simulink model "LPVattitudeLQRTracking"  (R2024b)
settings: Solver=ode45  StartTime=0.0  StopTime=tf  RelTol=1e-3
values from neighbouring files (symbols this model uses):
  gamma1_initial = deg2rad(0)    [CMG_Spacecraft_Attitude_Control.m]
  gamma2_initial = deg2rad(90)    [CMG_Spacecraft_Attitude_Control.m]
  p1 = linspace(gamma1_min,gamma1_max,gamma1_points)    [CMG_Spacecraft_Attitude_Control.m]
  p2 = linspace(gamma2_min,gamma2_max,gamma2_points)    [CMG_Spacecraft_Attitude_Control.m]
undefined symbols (not defined in the file or in its folder): K11, K12, K13, K14, K15, K16, K21, K22, K23, K24, K25, K26
libraries: simulink_extras x4, cstblocks x1
settings Model: PacingRate=1000  Creator=lanhi  LastModifiedBy=lanhi

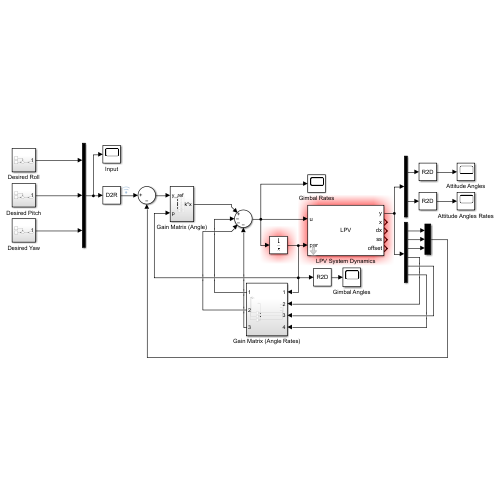
[thumbnail: Simulink's stored preview of the top-level diagram]
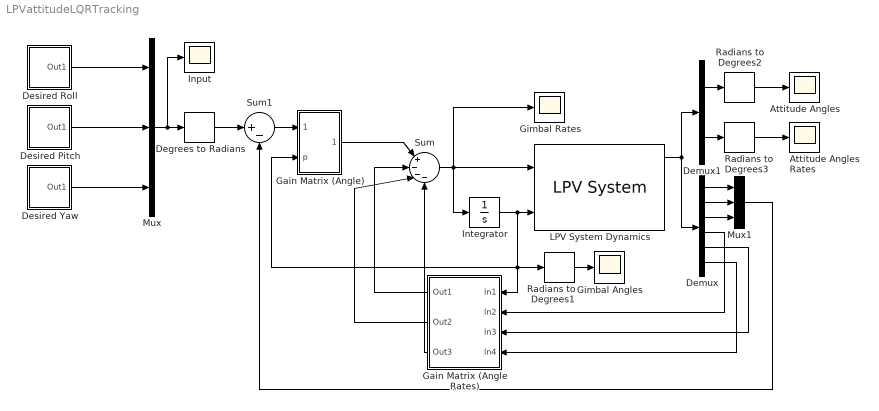
== system LPVattitudeLQRTracking ==
  Attitude Angles : Scope
  Attitude Angles Rates : Scope
  Degrees to Radians : simulink_extras/Transformations/Degrees to Radians
  Demux : Demux  Outputs=6
  Demux1 : Demux  Outputs=2
  Desired Pitch : Subsystem
  Desired Roll : Subsystem
  Desired Yaw : Subsystem
  Gain Matrix (Angle Rates) : Subsystem
  Gain Matrix (Angle) : Subsystem
  Gimbal Angles : Scope
  Gimbal Rates : Scope
  Input : Scope
  Integrator : Integrator  InitialCondition=[gamma1_initial,gamma2_initial]
  LPV System Dynamics : cstblocks/Linear Parameter Varying/LPV System  sys=ICs  InitialConditionSource=internal  InitialCondition=[deg2rad(0) deg2rad(0) deg2rad(0) deg2rad(0) deg2rad(0) deg2rad(0)]  opSpecOption=Specify offsets as double arrays  uOffset=0  yOffset=0  xOffset=0  opEquilOption=on  dxOffset=4  AFixed=false  BFixed=false  CFixed=false  DFixed=false  uDelayFixed=false  yDelayFixed=false  iDelayFixed=false  sysFixedOption=First model in state-space array  sysFixed=[]  IMethod=Linear  EMethod=Clip  IndexSearch=Binary search  IndexBegin=on  OutputX=on  OutputXdot=on  OutputLTI=on  OutputOP=on  DataType=double  InitBufferSize=1024  FixedBuffer=off  SimMode=Interpreted execution  Offset=struct
  Mux : Mux  Inputs=3
  Mux1 : Mux  Inputs=3
  Radians to Degrees1 : simulink_extras/Transformations/Radians to Degrees
  Radians to Degrees2 : simulink_extras/Transformations/Radians to Degrees
  Radians to Degrees3 : simulink_extras/Transformations/Radians to Degrees
  Sum : Sum  Inputs=|+---
  Sum1 : Sum  Inputs=|+-
  wires:
  Radians to Degrees1/1 -> Gimbal Angles/1
  LPV System Dynamics/1 -> Demux1/1, Demux/1
  Demux/1 -> Mux1/1
  Demux/2 -> Mux1/2
  Integrator/1 -> Gain Matrix (Angle Rates)/1(In1), Gain Matrix (Angle)/2(p), Radians to Degrees1/1, LPV System Dynamics/2
  Sum/1 -> Integrator/1, Gimbal Rates/1, LPV System Dynamics/1
  Gain Matrix (Angle)/1(k*x) -> Sum/1
  Mux/1 -> Degrees to Radians/1, Input/1
  Demux/3 -> Mux1/3
  Demux1/2 -> Radians to Degrees3/1
  Degrees to Radians/1 -> Sum1/1
  Sum1/1 -> Gain Matrix (Angle)/1(y_ref)
  Demux1/1 -> Radians to Degrees2/1
  Radians to Degrees2/1 -> Attitude Angles/1
  Radians to Degrees3/1 -> Attitude Angles Rates/1
  Mux1/1 -> Sum1/2
  Demux/4 -> Gain Matrix (Angle Rates)/2(In2)
  Demux/5 -> Gain Matrix (Angle Rates)/3(In3)
  Demux/6 -> Gain Matrix (Angle Rates)/4(In4)
  Gain Matrix (Angle Rates)/1(Out1) -> Sum/2
  Gain Matrix (Angle Rates)/2(Out2) -> Sum/3
  Gain Matrix (Angle Rates)/3(Out3) -> Sum/4
  Desired Roll/1(Out1) -> Mux/1
  Desired Pitch/1(Out1) -> Mux/2
  Desired Yaw/1(Out1) -> Mux/3

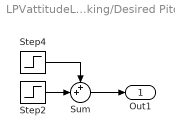
== system LPVattitudeLQRTracking/Desired Pitch ==
  Step2 : Step  Time=5  After=0  SampleTime=0
  Step4 : Step  After=0  SampleTime=0
  Sum : Sum  Inputs=++|
  Out1 : Outport
  wires:
  Step2/1 -> Sum/2
  Step4/1 -> Sum/1
  Sum/1 -> Out1/1

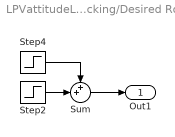
== system LPVattitudeLQRTracking/Desired Roll ==
  Step2 : Step  Time=5000  After=-15  SampleTime=0
  Step4 : Step  Time=1000  After=15  SampleTime=0
  Sum : Sum  Inputs=++|
  Out1 : Outport
  wires:
  Step2/1 -> Sum/2
  Step4/1 -> Sum/1
  Sum/1 -> Out1/1

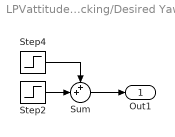
== system LPVattitudeLQRTracking/Desired Yaw ==
  Step2 : Step  Time=5  After=0  SampleTime=0
  Step4 : Step  After=0  SampleTime=0
  Sum : Sum  Inputs=++|
  Out1 : Outport
  wires:
  Step2/1 -> Sum/2
  Step4/1 -> Sum/1
  Sum/1 -> Out1/1

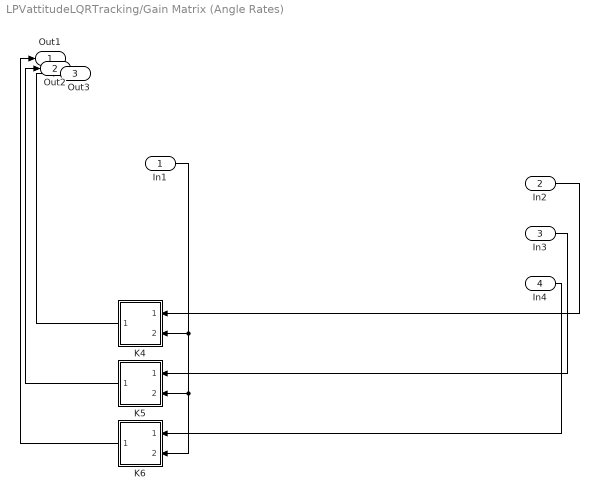
== system LPVattitudeLQRTracking/Gain Matrix (Angle Rates) ==
  In1 : Inport
  In2 : Inport  Port=2
  In3 : Inport  Port=3
  In4 : Inport  Port=4
  K4 : Subsystem
  K5 : Subsystem
  K6 : Subsystem
  Out1 : Outport
  Out2 : Outport  Port=2
  Out3 : Outport  Port=3
  wires:
  In2/1 -> K4/1(In1)
  K5/1(Out1) -> Out2/1
  In1/1 -> K6/2(In2), K5/2(In2), K4/2(In2)
  K6/1(Out1) -> Out1/1
  In4/1 -> K6/1(In1)
  K4/1(Out1) -> Out3/1
  In3/1 -> K5/1(In1)

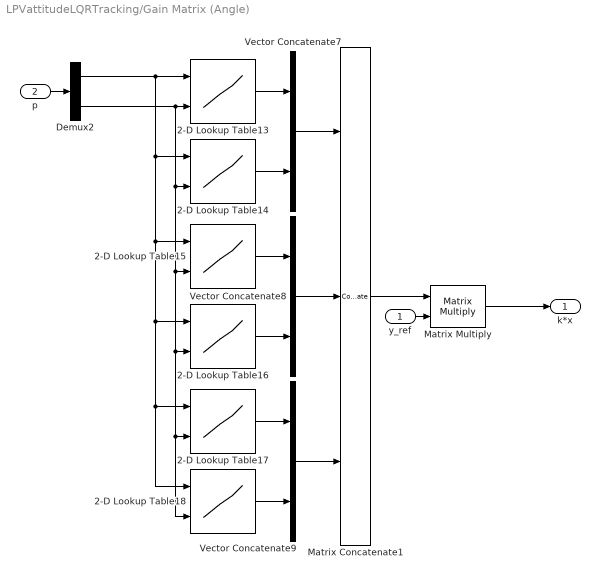
== system LPVattitudeLQRTracking/Gain Matrix (Angle) ==
  y_ref : Inport
  p : Inport  Port=2
  2-D Lookup Table13 : Lookup_n-D  BreakpointsForDimension1=p1  BreakpointsForDimension2=p2  Table=K11  InternalRulePriority=Speed  RndMeth=Simplest
      settings: InputPortMap=u0,u1
  2-D Lookup Table14 : Lookup_n-D  BreakpointsForDimension1=p1  BreakpointsForDimension2=p2  Table=K21  InternalRulePriority=Speed  RndMeth=Simplest
      settings: InputPortMap=u0,u1
  2-D Lookup Table15 : Lookup_n-D  BreakpointsForDimension1=p1  BreakpointsForDimension2=p2  Table=K12  InternalRulePriority=Speed  RndMeth=Simplest
      settings: InputPortMap=u0,u1
  2-D Lookup Table16 : Lookup_n-D  BreakpointsForDimension1=p1  BreakpointsForDimension2=p2  Table=K22  InternalRulePriority=Speed  RndMeth=Simplest
      settings: InputPortMap=u0,u1
  2-D Lookup Table17 : Lookup_n-D  BreakpointsForDimension1=p1  BreakpointsForDimension2=p2  Table=K13  InternalRulePriority=Speed  RndMeth=Simplest
      settings: InputPortMap=u0,u1
  2-D Lookup Table18 : Lookup_n-D  BreakpointsForDimension1=p1  BreakpointsForDimension2=p2  Table=K23  InternalRulePriority=Speed  RndMeth=Simplest
      settings: InputPortMap=u0,u1
  Demux2 : Demux  Outputs=2
  Matrix Concatenate1 : Concatenate  NumInputs=3  Mode=Multidimensional array  ConcatenateDimension=2
  Matrix Multiply : Product  Multiplication=Matrix(*)
  Vector Concatenate7 : Concatenate
  Vector Concatenate8 : Concatenate
  Vector Concatenate9 : Concatenate
  k*x : Outport
  wires:
  2-D Lookup Table14/1 -> Vector Concatenate7/2
  Demux2/1 -> 2-D Lookup Table13/1, 2-D Lookup Table14/1, 2-D Lookup Table15/1, 2-D Lookup Table16/1, 2-D Lookup Table17/1, 2-D Lookup Table18/1
  Vector Concatenate9/1 -> Matrix Concatenate1/3
  2-D Lookup Table15/1 -> Vector Concatenate8/1
  2-D Lookup Table16/1 -> Vector Concatenate8/2
  Demux2/2 -> 2-D Lookup Table18/2, 2-D Lookup Table17/2, 2-D Lookup Table16/2, 2-D Lookup Table15/2, 2-D Lookup Table14/2, 2-D Lookup Table13/2
  2-D Lookup Table13/1 -> Vector Concatenate7/1
  2-D Lookup Table17/1 -> Vector Concatenate9/1
  2-D Lookup Table18/1 -> Vector Concatenate9/2
  Vector Concatenate8/1 -> Matrix Concatenate1/2
  Vector Concatenate7/1 -> Matrix Concatenate1/1
  p/1 -> Demux2/1
  y_ref/1 -> Matrix Multiply/2
  Matrix Multiply/1 -> k*x/1
  Matrix Concatenate1/1 -> Matrix Multiply/1

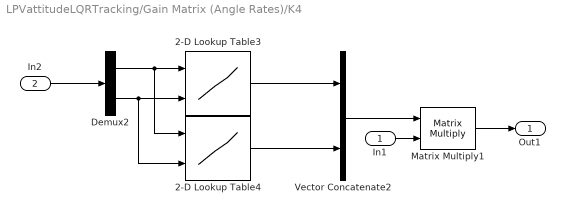
== system LPVattitudeLQRTracking/Gain Matrix (Angle Rates)/K4 ==
  In1 : Inport
  In2 : Inport  Port=2
  2-D Lookup Table3 : Lookup_n-D  BreakpointsForDimension1=p1  BreakpointsForDimension2=p2  Table=K14  InternalRulePriority=Speed  RndMeth=Simplest
      settings: InputPortMap=u0,u1
  2-D Lookup Table4 : Lookup_n-D  BreakpointsForDimension1=p1  BreakpointsForDimension2=p2  Table=K24  InternalRulePriority=Speed  RndMeth=Simplest
      settings: InputPortMap=u0,u1
  Demux2 : Demux  Outputs=2
  Matrix Multiply1 : Product  Multiplication=Matrix(*)
  Vector Concatenate2 : Concatenate
  Out1 : Outport
  wires:
  Demux2/1 -> 2-D Lookup Table4/1, 2-D Lookup Table3/1
  Demux2/2 -> 2-D Lookup Table4/2, 2-D Lookup Table3/2
  2-D Lookup Table4/1 -> Vector Concatenate2/2
  2-D Lookup Table3/1 -> Vector Concatenate2/1
  Vector Concatenate2/1 -> Matrix Multiply1/1
  Matrix Multiply1/1 -> Out1/1
  In2/1 -> Demux2/1
  In1/1 -> Matrix Multiply1/2

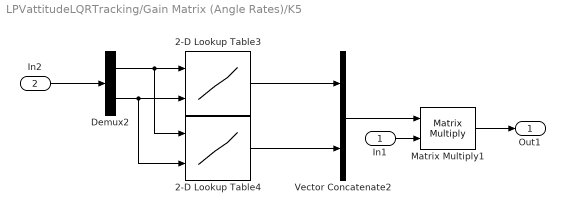
== system LPVattitudeLQRTracking/Gain Matrix (Angle Rates)/K5 ==
  In1 : Inport
  In2 : Inport  Port=2
  2-D Lookup Table3 : Lookup_n-D  BreakpointsForDimension1=p1  BreakpointsForDimension2=p2  Table=K15  InternalRulePriority=Speed  RndMeth=Simplest
      settings: InputPortMap=u0,u1
  2-D Lookup Table4 : Lookup_n-D  BreakpointsForDimension1=p1  BreakpointsForDimension2=p2  Table=K25  InternalRulePriority=Speed  RndMeth=Simplest
      settings: InputPortMap=u0,u1
  Demux2 : Demux  Outputs=2
  Matrix Multiply1 : Product  Multiplication=Matrix(*)
  Vector Concatenate2 : Concatenate
  Out1 : Outport
  wires:
  Demux2/1 -> 2-D Lookup Table4/1, 2-D Lookup Table3/1
  Demux2/2 -> 2-D Lookup Table4/2, 2-D Lookup Table3/2
  2-D Lookup Table4/1 -> Vector Concatenate2/2
  2-D Lookup Table3/1 -> Vector Concatenate2/1
  Vector Concatenate2/1 -> Matrix Multiply1/1
  Matrix Multiply1/1 -> Out1/1
  In2/1 -> Demux2/1
  In1/1 -> Matrix Multiply1/2

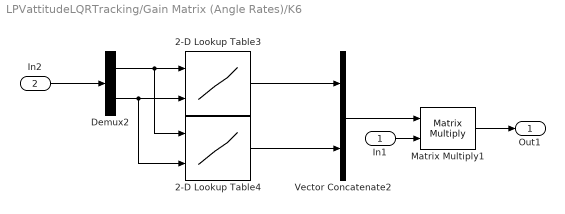
== system LPVattitudeLQRTracking/Gain Matrix (Angle Rates)/K6 ==
  In1 : Inport
  In2 : Inport  Port=2
  2-D Lookup Table3 : Lookup_n-D  BreakpointsForDimension1=p1  BreakpointsForDimension2=p2  Table=K16  InternalRulePriority=Speed  RndMeth=Simplest
      settings: InputPortMap=u0,u1
  2-D Lookup Table4 : Lookup_n-D  BreakpointsForDimension1=p1  BreakpointsForDimension2=p2  Table=K26  InternalRulePriority=Speed  RndMeth=Simplest
      settings: InputPortMap=u0,u1
  Demux2 : Demux  Outputs=2
  Matrix Multiply1 : Product  Multiplication=Matrix(*)
  Vector Concatenate2 : Concatenate
  Out1 : Outport
  wires:
  Demux2/1 -> 2-D Lookup Table4/1, 2-D Lookup Table3/1
  Demux2/2 -> 2-D Lookup Table4/2, 2-D Lookup Table3/2
  2-D Lookup Table4/1 -> Vector Concatenate2/2
  2-D Lookup Table3/1 -> Vector Concatenate2/1
  Vector Concatenate2/1 -> Matrix Multiply1/1
  Matrix Multiply1/1 -> Out1/1
  In2/1 -> Demux2/1
  In1/1 -> Matrix Multiply1/2
